simulink model "second_order_integrator"  (R2023a)
settings: Solver=VariableStepAuto  StartTime=0.0  StopTime=30  RelTol=1e-3
undefined symbols (not defined in the file or in its folder): wn
settings Model: Creator=Adan Daniel  LastModifiedBy=Adan Daniel

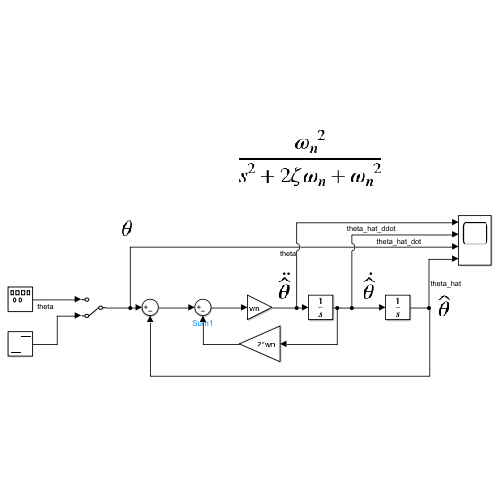
[thumbnail: Simulink's stored preview of the top-level diagram]
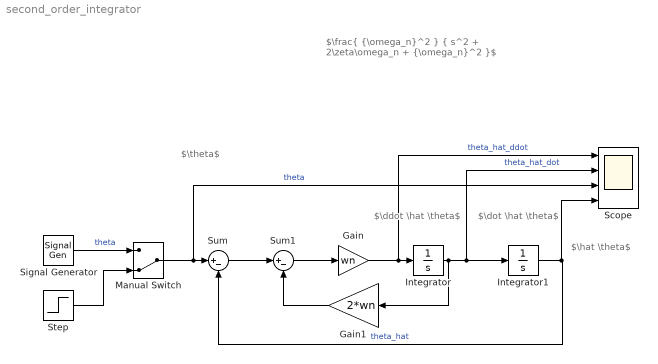
== system second_order_integrator ==
  note: $\theta$
  note: $\frac{ {\omega_n}^2 } { s^2 + 2\zeta\omega_n + {\omega_n}^2 }$
  note: $\ddot \hat \theta$
  note: $\dot \hat \theta$
  note: $\hat \theta$
  Gain : Gain  Gain=wn
  Gain1 : Gain  Gain=2*wn
  Integrator : Integrator
  Integrator1 : Integrator
  Manual Switch : ManualSwitch  CurrentSetting=0
  Scope : Scope  NumInputPorts=4
  Signal Generator : SignalGenerator  Amplitude=0.1  Units=rad/sec
  Step : Step  After=0.1  SampleTime=0
  Sum : Sum  Inputs=|+-
  Sum1 : Sum  Inputs=|+-
  wires:
  Signal Generator/1 -> Manual Switch/1  "theta"
  Sum/1 -> Sum1/1
  Sum1/1 -> Gain/1
  Gain/1 -> Scope/1, Integrator/1  "theta_hat_ddot"
  Integrator/1 -> Gain1/1, Scope/2, Integrator1/1  "theta_hat_dot"
  Gain1/1 -> Sum1/2
  Integrator1/1 -> Scope/4, Sum/2  "theta_hat"
  Manual Switch/1 -> Scope/3, Sum/1  "theta"
  Step/1 -> Manual Switch/2
